simulink model "Exemplu_figura9"  (R2016a)
settings: Solver=VariableStepDiscrete  StartTime=0.0  StopTime=500  RelTol=1e-3
undefined symbols (not defined in the file): entity, f, m, n
settings Model: Creator=Cristina  LastModifiedBy=Cristina

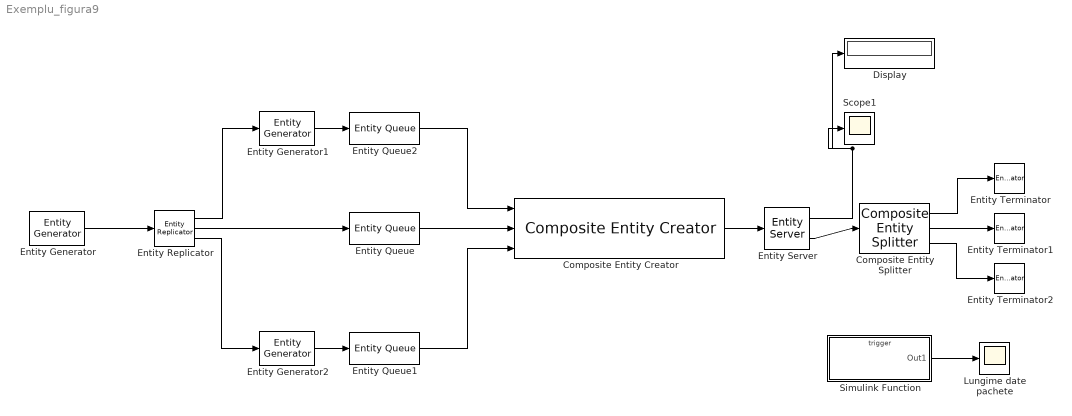
== system Exemplu_figura9 ==
  Composite Entity Creator : CompositeEntityCreator  InputPortMessageModes=m,m,m  OutputPortMessageModes=m  NumberInputPorts=3  EntityTypeName=Combined  InputEntityName=HeaderLength|PayloadLength|TrailerLength
      settings: InputPortMap=u0,u1,u2
  Composite Entity Splitter : CompositeEntitySplitter  InputPortMessageModes=m  OutputPortMessageModes=m,m,m  NumberOutputPorts=3
      settings: OutputPortMap=o0,o1,o2
  Display : Display
  Entity Generator : EntityGenerator  OutputPortMessageModes=m  TimeSource=MATLAB action  IntergenerationTimeAction=|  GenerateAction=|  AttributeName=PayloadLength|Length  AttributeInitialValue=1|0  EntityType=Structured  EntityTypeName=Payload
      IntergenerationTimeAction=|
      | persistent init
      | if (isempty(init))
      |     init = true;
      |     rng(23795);
      | end
      | dt = exprnd(1);
      GenerateAction=|
      | persistent x
      | 
      | if (isempty(x))
      |     rng(86493);
      |     x = true;
      | end
      | entity.PayloadLength = randi([10,1500]);
  Entity Generator1 : EntityGenerator  InputPortMessageModes=m  OutputPortMessageModes=m  GenerationMethod=Event-based  AttributeName=HeaderLength  AttributeInitialValue=14  EntityType=Structured  EntityTypeName=Header
      settings: InputPortMap=u0
  Entity Generator2 : EntityGenerator  InputPortMessageModes=m  OutputPortMessageModes=m  GenerationMethod=Event-based  AttributeName=TrailerLength  AttributeInitialValue=4  EntityType=Structured  EntityTypeName=Trailer
      settings: InputPortMap=u0
  Entity Queue : EntityQueue  InputPortMessageModes=m  OutputPortMessageModes=m
      settings: OutputPortMap=o5
  Entity Queue1 : EntityQueue  InputPortMessageModes=m  OutputPortMessageModes=m
      settings: OutputPortMap=o5
  Entity Queue2 : EntityQueue  InputPortMessageModes=m  OutputPortMessageModes=m
      settings: OutputPortMap=o5
  Entity Replicator : EntityReplicator  InputPortMessageModes=m  OutputPortMessageModes=m,m,m  NumberReplicas=2
      settings: OutputPortMap=o0,o1,o2
  Entity Server : EntityServer  InputPortMessageModes=m  OutputPortMessageModes=n,m  Capacity=1  EntryAction=|  NumberEntitiesDeparted=on
      | entity.PayloadLength.Length = ...
      |     (entity.HeaderLength.HeaderLength + ...
      |     entity.PayloadLength.PayloadLength + ...
      |     entity.TrailerLength.TrailerLength) * 0.001;
      settings: OutputPortMap=o0,o9
  Entity Terminator : EntityTerminator  InputPortMessageModes=m
  Entity Terminator1 : EntityTerminator  InputPortMessageModes=m  EntryAction=f(entity.PayloadLength);
  Entity Terminator2 : EntityTerminator  InputPortMessageModes=m
  Lungime date pachete : Scope
  Scope1 : Scope
  Simulink Function : Subsystem  TreatAsAtomicUnit=on
  wires:
  Entity Generator/1 -> Entity Replicator/1
  Entity Replicator/1 -> Entity Generator1/1
  Entity Replicator/3 -> Entity Generator2/1
  Entity Replicator/2 -> Entity Queue/1
  Entity Generator2/1 -> Entity Queue1/1
  Entity Generator1/1 -> Entity Queue2/1
  Entity Queue2/1 -> Composite Entity Creator/1
  Entity Queue/1 -> Composite Entity Creator/2
  Entity Queue1/1 -> Composite Entity Creator/3
  Composite Entity Creator/1 -> Entity Server/1
  Entity Server/2 -> Composite Entity Splitter/1
  Composite Entity Splitter/1 -> Entity Terminator/1
  Composite Entity Splitter/3 -> Entity Terminator2/1
  Composite Entity Splitter/2 -> Entity Terminator1/1
  Simulink Function/1(Out1) -> Lungime date pachete/1
  Entity Server/1 -> Display/1, Scope1/1

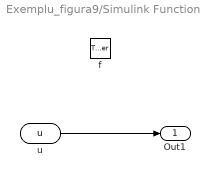
== system Exemplu_figura9/Simulink Function ==
  f : TriggerPort  TriggerType=function-call  IsSimulinkFunction=on  FunctionName=f  VariantControl=Variant
  u : ArgIn  DisableCoverage=on  ArgumentName=u
  Out1 : Outport
  wires:
  u/1 -> Out1/1
